simulink model "s4_MDL_Tlepkie_lqi_dol"  (R2023a)
settings: Solver=ode4  StartTime=0.0  StopTime=end_time  FixedStep=dt  MaxStep=0.001  RelTol=1e-3
values from neighbouring files (symbols this model uses):
  dt = 0.001    [anim_sim_script.m]    (also in s3_lqr_Dol_simulink.m; s4_LQI_Dol_simulink.m)
  K = lqr(A, B, Q, R)    [s2_lqr_Dol_tylko_skrypt.m]    (also in s3_lqr_Dol_simulink.m; s4_LQI_Dol_simulink.m = lqr(Aa, Ba, Q, R))
  PP = [track_len/2; pi; 0; 0]    [s3_lqr_Dol_simulink.m]    (also in s4_LQI_Dol_simulink.m)
  track_len = 0.47    [anim_sim_script.m]    (also in s3_lqr_Dol_simulink.m; s4_LQI_Dol_simulink.m)
  x0NL = [ ... (first row only)    [s3_lqr_Dol_simulink.m]    (also in s4_LQI_Dol_simulink.m)
settings Model: Creator=Adam  LastModifiedBy=Adam
settings SolverCC: AlgebraicLoopSolver=TrustRegion
settings DataIOCC: SaveOutput=off  SignalLogging=off  DSMLogging=off
settings DebuggingCC: AlgebraicLoopMsg=none  UnconnectedInputMsg=warning  UnconnectedOutputMsg=warning  UnconnectedLineMsg=warning
settings ModelReferenceCC: EnableRefExpFcnMdlSchedulingChecks=on
settings RTWCC: DLArmComputeVersion=19.05

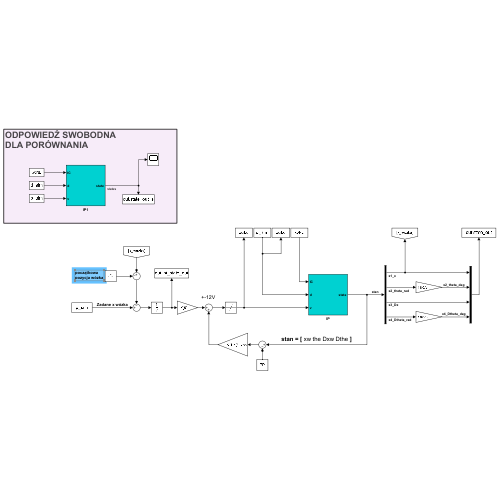
[thumbnail: Simulink's stored preview of the top-level diagram]
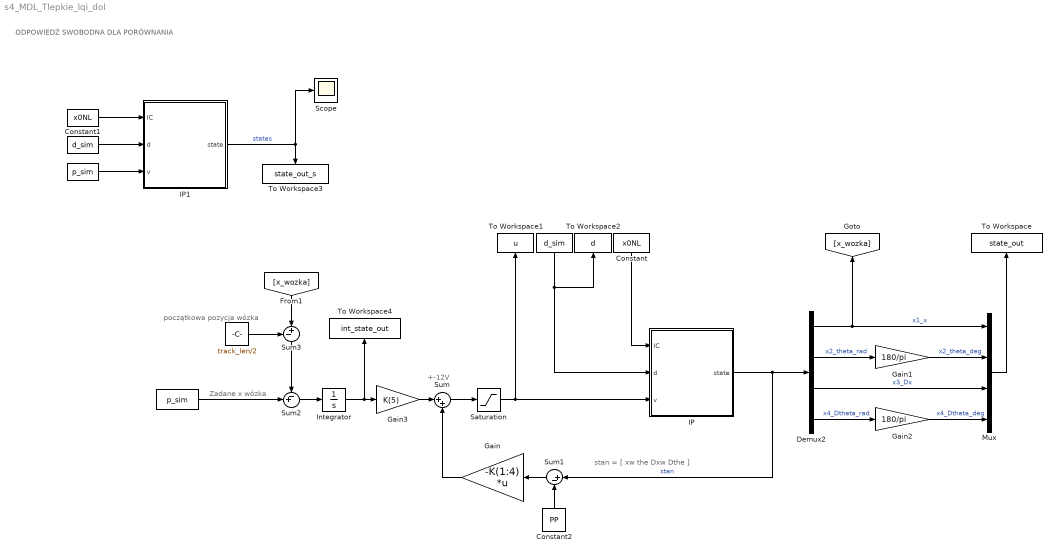
== system s4_MDL_Tlepkie_lqi_dol ==
  note: ODPOWIEDŹ SWOBODNA
      | DLA PORÓWNANIA
  note: stan = [ xw the Dxw Dthe ]
  note: Zadane x wózka
  note: +-12V
  note: początkowa
      | pozycja wózka
  " " : FromWorkspace  VariableName=p_sim  SampleTime=dt
  "  " : FromWorkspace  VariableName=d_sim  SampleTime=dt
  "   " : FromWorkspace  VariableName=d_sim  SampleTime=dt
  "      " : FromWorkspace  VariableName=p_sim  SampleTime=dt
  "       " : Constant  Value=track_len/2
  Constant : Constant  Value=x0NL
  Constant1 : Constant  Value=x0NL
  Constant2 : Constant  Value=PP
  Demux2 : Demux
  Gain : Gain  Gain=-K(1:4)  Multiplication=Matrix(K*u) (u vector)
  Gain1 : Gain  Gain=180/pi
  Gain2 : Gain  Gain=180/pi
  Gain3 : Gain  Gain=K(5)
  IP : Subsystem
  IP1 : Subsystem
  Integrator : Integrator
  Mux : Mux
  Saturation : Saturate  UpperLimit=12  LowerLimit=-12
  Scope : Scope
  Sum : Sum  Inputs=|++
  Sum1 : Sum  Inputs=|+-
  Sum2 : Sum  Inputs=-+|
  Sum3 : Sum  Inputs=-+|
  To Workspace : ToWorkspace  VariableName=state_out  SampleTime=-1
  To Workspace1 : ToWorkspace  VariableName=u  SampleTime=-1
  To Workspace2 : ToWorkspace  VariableName=d  SampleTime=-1
  To Workspace3 : ToWorkspace  VariableName=state_out_s  SampleTime=-1
  To Workspace4 : ToWorkspace  VariableName=int_state_out  SampleTime=-1
  wires:
  Gain2/1 -> Mux/4  "x4_Dtheta_deg"
  Demux2/4 -> Gain2/1  "x4_Dtheta_rad"
  Demux2/3 -> Mux/3  "x3_Dx"
  Demux2/2 -> Gain1/1  "x2_theta_rad"
  Demux2/1 -> Mux/1, [x_wozka]  "x1_x"
  Gain1/1 -> Mux/2  "x2_theta_deg"
  IP/1(state) -> Sum1/1, Demux2/1  "stan"
  Constant/1 -> IP/1(IC)
  Saturation/1 -> IP/3(v), To Workspace1/1
  Mux/1 -> To Workspace/1
  "  "/1 -> To Workspace2/1, IP/2(d)
  Constant1/1 -> IP1/1(IC)
  "   "/1 -> IP1/2(d)
  Sum/1 -> Saturation/1
  Gain/1 -> Sum/2
  "      "/1 -> IP1/3(v)
  IP1/1(state) -> To Workspace3/1, Scope/1  "states"
  Sum1/1 -> Gain/1
  Constant2/1 -> Sum1/2
  Integrator/1 -> To Workspace4/1, Gain3/1
  Sum2/1 -> Integrator/1
  Gain3/1 -> Sum/1
  " "/1 -> Sum2/2
  [x_wozka] -> Sum3/2
  Sum3/1 -> Sum2/1
  "       "/1 -> Sum3/1

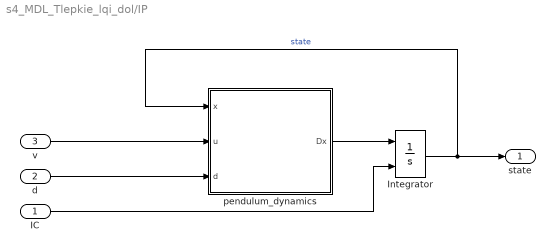
== system s4_MDL_Tlepkie_lqi_dol/IP ==
  IC : Inport
  d : Inport  Port=2
  v : Inport  Port=3
  Integrator : Integrator  InitialConditionSource=external
  pendulum_dynamics : MATLAB Function  TreatAsAtomicUnit=on
  state : Outport
  wires:
  Integrator/1 -> state/1, pendulum_dynamics/1(x)  "state"
  v/1 -> pendulum_dynamics/2(u)
  pendulum_dynamics/1(Dx) -> Integrator/1
  IC/1 -> Integrator/2
  d/1 -> pendulum_dynamics/3(d)

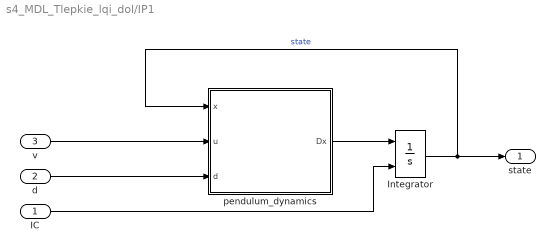
== system s4_MDL_Tlepkie_lqi_dol/IP1 ==
  IC : Inport
  d : Inport  Port=2
  v : Inport  Port=3
  Integrator : Integrator  InitialConditionSource=external
  pendulum_dynamics : MATLAB Function  TreatAsAtomicUnit=on
  state : Outport
  wires:
  Integrator/1 -> state/1, pendulum_dynamics/1(x)  "state"
  v/1 -> pendulum_dynamics/2(u)
  pendulum_dynamics/1(Dx) -> Integrator/1
  IC/1 -> Integrator/2
  d/1 -> pendulum_dynamics/3(d)

== matlab function s4_MDL_Tlepkie_lqi_dol/IP1/pendulum_dynamics ==
  data: x input; u input; d input; Dx output; params_lepkie parameter
function Dx = dynamika_wahadla(x, u, d, params_lepkie)
% x : stan
% u : input - napięcie
%
% params scope: "parameters"
%

% State, function input: x = [x Dx theta Dtheta]'
x1 = x(1);
x2 = x(2); 
x3 = x(3);
x4 = x(4);

params_lepkie = num2cell(params_lepkie);
[M, mc, mp, Lp, Lc, g, b, gamma, mr, Mt, L, Jcm, Jt, alpha, beta] = params_lepkie{:};

% Equations for pendulum dynamics
Ff = b*x3;
Fi = alpha*u - beta*x3;
A = d*cos(x2) - Ff + L*mr*x4^2*sin(x2) + Fi;
B = d*Lc + L*g*mr*sin(x2) - gamma*x4;
DEN = Jt*Mt - (L*mr*cos(x2))^2;

ddt_x1 = x3;
ddt_x2 = x4;
ddt_x3 = (Jt*A - L*mr*cos(x2)*B) / DEN;
ddt_x4 = (Mt*B - L*mr*cos(x2)*A) / DEN;

% output
Dx = [ddt_x1 ddt_x2 ddt_x3 ddt_x4]';

end

== matlab function s4_MDL_Tlepkie_lqi_dol/IP/pendulum_dynamics ==
  data: x input; u input; d input; Dx output; params_lepkie parameter
function Dx = dynamika_wahadla(x, u, d, params_lepkie)
% x : stan
% u : input - napięcie
%
% params scope: "parameters"
%

% State, function input: x = [x Dx theta Dtheta]'
x1 = x(1);
x2 = x(2); 
x3 = x(3);
x4 = x(4);

params_lepkie = num2cell(params_lepkie);
[M, mc, mp, Lp, Lc, g, b, gamma, mr, Mt, L, Jcm, Jt, alpha, beta] = params_lepkie{:};

% Equations for pendulum dynamics
Ff = b*x3;
Fi = alpha*u - beta*x3;
A = d*cos(x2) - Ff + L*mr*x4^2*sin(x2) + Fi;
B = d*Lc + L*g*mr*sin(x2) - gamma*x4;
DEN = Jt*Mt - (L*mr*cos(x2))^2;

ddt_x1 = x3;
ddt_x2 = x4;
ddt_x3 = (Jt*A - L*mr*cos(x2)*B) / DEN;
ddt_x4 = (Mt*B - L*mr*cos(x2)*A) / DEN;

% output
Dx = [ddt_x1 ddt_x2 ddt_x3 ddt_x4]';

end
